simulink model "Randomised_Algorithm_Quadcopter_Simulation"  (R2017a)
settings: Solver=ode45  StartTime=0.0  StopTime=35  FixedStep=0.05  MaxStep=0.06  RelTol=1e-3  EnableMultiTasking=on
model workspace (MAT data in the model file):
  MCOS : class17 (value not decoded)
undefined symbols (not defined in the file or in its folder): altitude_error, error1, error2, error3, error4, IC, quadModel
libraries: simulink x4
(part 2 of 2)

== matlab function Randomised_Algorithm_Quadcopter_Simulation/Quadcopter Dynamics/Motor Dynamics/Subsystem1/MATLAB Function ==
  data: fault input; nominal_modal_input input; rotor_speed output
function rotor_speed = fcn(  fault, nominal_modal_input)


rotor_speed =  (nominal_modal_input* (1-fault));

end

== matlab function Randomised_Algorithm_Quadcopter_Simulation/Position Controller/MATLAB Function ==
  data: y_error input; x_error input; max_error_signal data_store_memory; count data_store_memory; time input; prevTime data_store_memory
function fcn(y_error,x_error,time)
global prevTime;
global max_error_signal;
global count;
%if(abs(y_error) + abs(x_error) > max_error_signal)
if(prevTime+0.1 < time)
    max_error_signal = max_error_signal + abs(y_error) + abs(x_error);
    count =count +1;
    %disp(count);
    prevTime = time;
end
end

== matlab function Randomised_Algorithm_Quadcopter_Simulation/Quadcopter Dynamics/Motor Dynamics/Subsystem2/MATLAB Function ==
  data: fault input; nominal_modal_input input; rotor_speed output
function rotor_speed = fcn(  fault, nominal_modal_input)


rotor_speed =  (nominal_modal_input* (1-fault));

end

== matlab function Randomised_Algorithm_Quadcopter_Simulation/Quadcopter Dynamics/Motor Dynamics/Subsystem3/MATLAB Function ==
  data: fault input; nominal_modal_input input; rotor_speed output
function rotor_speed = fcn(  fault, nominal_modal_input)


rotor_speed =  (nominal_modal_input* (1-fault));

end

== matlab function Randomised_Algorithm_Quadcopter_Simulation/Attitude Controller/blending 1 ==
  data: control_signal output; portion input; fault_controller input; nominal_controller input
function control_signal = blending(portion , fault_controller, nominal_controller)

fault_part = (fault_controller * portion);
nominal_portion = 1-portion;
nominal_part = nominal_controller * nominal_portion;
control_signal = fault_part + nominal_part;

end

== matlab function Randomised_Algorithm_Quadcopter_Simulation/Attitude Controller/blending 2 ==
  data: control_signal output; portion input; fault_controller input; nominal_controller input
function control_signal = blending(portion , fault_controller, nominal_controller)

fault_part = (fault_controller * portion);
nominal_portion = 1-portion;
nominal_part = nominal_controller * nominal_portion;
control_signal = fault_part + nominal_part;

end

== matlab function Randomised_Algorithm_Quadcopter_Simulation/Attitude Controller/High Level Randomised Algorithm ==
  data: current_error input; Phi output; Theta output; Psi output; previousTime data_store_memory; blend data_store_memory; time input; Phi_blend data_store_memory; Theta_blend data_store_memory; Psi_blend data_store_memory; count output
function [Phi, Theta, Psi, count]= fcn(current_error, time)

%global lookup_table;
global previousTime;
%current_error_index = (current_error*1000) +1;
global Phi_blend;
global Theta_blend;
global Psi_blend;

%if(previousTime < time)
Psi_blend = Psi_blend +1;
count = Psi_blend;
    if(current_error > 0)
        %stored_value = lookup_table(current_error_index);
        %if( stored_value == -1)
        %generate random blend
        blend = rand();
        %blend = 0;
        Phi = blend;
        Theta= blend;
        Psi = blend;
        
        Phi_blend = blend;
        Theta_blend =blend;
        Psi_blend = Phi_blend;
        %   lookup_table(current_error_index) = blend;
     
    else
        Phi = 0;
        Theta = 0;
        Psi = 0;
        
    end
%else
  %  Phi = Phi_blend;
  %  Theta= Theta_blend;
   % Psi = Psi_blend;
%end

%previousTime = time;

== matlab function Randomised_Algorithm_Quadcopter_Simulation/Position Controller/MATLAB Function1 ==
  data: alt_diff input; y output; altitude_error data_store_memory; time input; PrevTime2 data_store_memory
function y = fcn(alt_diff, time)
global altitude_error;
global PrevTime2;

if(PrevTime2+0.1 < time)
    altitude_error = altitude_error + abs(alt_diff);

    y = altitude_error;
    PrevTime2 = time;
else
    y = altitude_error;
end
